simulink model "Taller_2"  (R2025b)
settings: Solver=VariableStepAuto  StartTime=0.0  StopTime=5  RelTol=1e-3
libraries: simulink x7
settings Model: Creator=andre  LastModifiedBy=andre

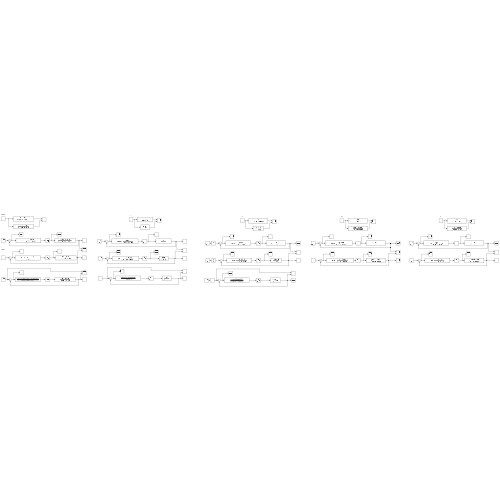
[thumbnail: Simulink's stored preview of the top-level diagram]
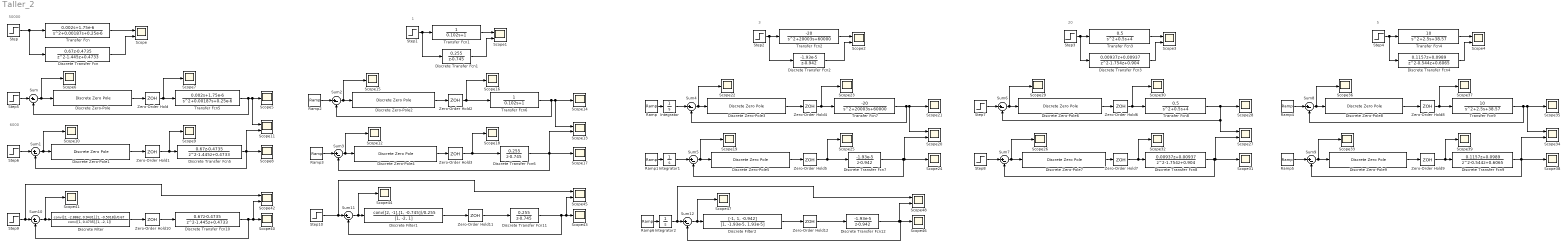
== system Taller_2 ==
  note: 1
  note: 50000
  note: 3
  note: 20
  note: 5
  note: 6000
  Discrete Transfer Fcn : DiscreteTransferFcn  Numerator=[0.67 -0.4735]  Denominator=[1 -1.445 0.4733]
  Discrete Transfer Fcn1 : DiscreteTransferFcn  Numerator=[0.255]  Denominator=[1 -0.745]
  Discrete Transfer Fcn10 : DiscreteTransferFcn  Numerator=[0.67 -0.4735]  Denominator=[1 -1.445 0.4733]
  Discrete Transfer Fcn11 : DiscreteTransferFcn  Numerator=[0.255]  Denominator=[1 -0.745]
  Discrete Transfer Fcn12 : DiscreteTransferFcn  Numerator=[-1.93e-5]  Denominator=[1 -0.942]
  Discrete Transfer Fcn2 : DiscreteTransferFcn  Numerator=[-1.93e-5]  Denominator=[1 -0.942]
  Discrete Transfer Fcn3 : DiscreteTransferFcn  Numerator=[0.00937 0.00937]  Denominator=[1 -1.754 0.904]
  Discrete Transfer Fcn4 : DiscreteTransferFcn  Numerator=[0.1157 0.0989]  Denominator=[1 -0.544 0.6065]
  Discrete Transfer Fcn5 : DiscreteTransferFcn  Numerator=[0.67 -0.4735]  Denominator=[1 -1.445 0.4733]
  Discrete Transfer Fcn6 : DiscreteTransferFcn  Numerator=[0.255]  Denominator=[1 -0.745]
  Discrete Transfer Fcn7 : DiscreteTransferFcn  Numerator=[-1.93e-5]  Denominator=[1 -0.942]
  Discrete Transfer Fcn8 : DiscreteTransferFcn  Numerator=[0.00937 0.00937]  Denominator=[1 -1.754 0.904]
  Discrete Transfer Fcn9 : DiscreteTransferFcn  Numerator=[0.1157 0.0989]  Denominator=[1 -0.544 0.6065]
  Discrete Zero-Pole : DiscreteZeroPole  Zeros=[0.9432 0.9432 0.9432]  Poles=[1 0.7364 0.7364 0.7364]  Gain=3.25e-4  SampleTime=400
  Discrete Zero-Pole1 : DiscreteZeroPole  Zeros=[0.9432 0.9432 0.9432]  Poles=[1 0.7364 0.7364 0.7364]  Gain=3.25e-4  SampleTime=400
  Discrete Zero-Pole2 : DiscreteZeroPole  Zeros=[0.745 0.745 0.745]  Poles=[1 1 0.6749 0.6749 0.6749]  Gain=1.031e-2  SampleTime=0.05
  Discrete Zero-Pole3 : DiscreteZeroPole  Zeros=[0.942 0.942 0.942]  Poles=[1 1 1 0.936 0.936 0.936]  Gain=-0.0433  SampleTime=0.02
  Discrete Zero-Pole4 : DiscreteZeroPole  Zeros=[0.745 0.745 0.745]  Poles=[1 1 0.6749 0.6749 0.6749]  Gain=1.031e-2  SampleTime=0.05
  Discrete Zero-Pole5 : DiscreteZeroPole  Zeros=[0.942 0.942 0.942]  Poles=[1 1 1 0.936 0.936 0.936]  Gain=-0.0433  SampleTime=0.02
  Discrete Zero-Pole6 : DiscreteZeroPole  Zeros=[0.9549 0.9549 0.9549]  Poles=[1 1 0.9581 0.9581 0.9581]  Gain=0.01468  SampleTime=0.2
  Discrete Zero-Pole7 : DiscreteZeroPole  Zeros=[0.9549 0.9549 0.9549]  Poles=[1 1 0.9581 0.9581 0.9581]  Gain=0.01468  SampleTime=0.2
  Discrete Zero-Pole8 : DiscreteZeroPole  Zeros=[0.717 0.717]  Poles=[1 1 0.952 0.952]  Gain=3.75  SampleTime=0.2
  Discrete Zero-Pole9 : DiscreteZeroPole  Zeros=[0.717 0.717]  Poles=[1 1 0.952 0.952]  Gain=3.75  SampleTime=0.2
  Discrete Filter : DiscreteFilter  Numerator=conv([2, -2.8862, 0.9431],[1, -0.5018])/0.67  Denominator=conv([1, 0.4735],[1, -2, 1])
  Discrete Filter1 : DiscreteFilter  Numerator=conv([2, -1],[1, -0.745])/0.255  Denominator=[1, -2, 1]
  Discrete Filter2 : DiscreteFilter  Numerator=[-1, 1, -0.942]  Denominator=[1, -1.93e-5, 1.93e-5]
  Integrator : Integrator
  Integrator1 : Integrator
  Integrator2 : Integrator
  Ramp{,1..6} (7 alike) : simulink/Sources/Ramp  slope=1  start=0  InitialOutput=0
  Scope{,1..4,11,13,20,27,34,42,45,48} (13 alike) : Scope  NumInputPorts=2
      Scope settings: ActiveDisplayYMinimum=-0.87443172150614323  ActiveDisplayYMaximum=7.8698854935552909
      Scope1 settings: ActiveDisplayYMinimum=-0.12499999999997945  ActiveDisplayYMaximum=1.1249999999998153
      Scope11 settings: ActiveDisplayYMinimum=-1  ActiveDisplayYMaximum=1  DataLoggingVariableName=ScopeData11
      Scope13 settings: ActiveDisplayYMinimum=-1  ActiveDisplayYMaximum=1  DataLoggingVariableName=ScopeData13
      Scope2 settings: ActiveDisplayYMinimum=-0.0003749537356942865  ActiveDisplayYMaximum=4.1661526188254047E-5  DataLoggingVariableName=ScopeData2
      Scope20 settings: ActiveDisplayYMinimum=-1  ActiveDisplayYMaximum=1  DataLoggingVariableName=ScopeData20
      Scope27 settings: ActiveDisplayYMinimum=-1  ActiveDisplayYMaximum=1  DataLoggingVariableName=ScopeData27
      Scope3 settings: ActiveDisplayYMinimum=-0.026140229104854404  ActiveDisplayYMaximum=0.2352620619436897  DataLoggingVariableName=ScopeData3
      Scope34 settings: ActiveDisplayYMinimum=-16759.782546183404  ActiveDisplayYMaximum=10006.031814391354  DataLoggingVariableName=ScopeData34
      Scope4 settings: ActiveDisplayYMinimum=-0.049373131397526727  ActiveDisplayYMaximum=0.44435818257774068  DataLoggingVariableName=ScopeData4
      Scope42 settings: ActiveDisplayYMinimum=-11114.4553559121  ActiveDisplayYMaximum=19001.265185022872  DataLoggingVariableName=ScopeData42
      Scope45 settings: ActiveDisplayYMinimum=-2.5344855037279E+9  ActiveDisplayYMaximum=9.5632271965801024E+8  DataLoggingVariableName=ScopeData45
      Scope48 settings: ActiveDisplayYMinimum=-0.56305934372930366  ActiveDisplayYMaximum=5.0675340935637339  DataLoggingVariableName=ScopeData48
  Scope{5..10,12,14..19,21..26,28..33,35..41,43..44,46..47} (36 alike) : Scope
      Scope10 settings: DataLoggingVariableName=ScopeData10
      Scope12 settings: ActiveDisplayYMinimum=-1  ActiveDisplayYMaximum=1  DataLoggingVariableName=ScopeData12
      Scope14 settings: ActiveDisplayYMinimum=-1  ActiveDisplayYMaximum=1  DataLoggingVariableName=ScopeData14
      Scope15 settings: ActiveDisplayYMinimum=-0.11913455922896504  ActiveDisplayYMaximum=1.0722110330606855  DataLoggingVariableName=ScopeData15
      Scope16 settings: ActiveDisplayYMinimum=-1  ActiveDisplayYMaximum=1  DataLoggingVariableName=ScopeData16
      Scope17 settings: ActiveDisplayYMinimum=-1  ActiveDisplayYMaximum=1  DataLoggingVariableName=ScopeData17
      Scope18 settings: ActiveDisplayYMinimum=-1  ActiveDisplayYMaximum=1  DataLoggingVariableName=ScopeData18
      Scope19 settings: ActiveDisplayYMinimum=-1  ActiveDisplayYMaximum=1  DataLoggingVariableName=ScopeData19
      Scope21 settings: ActiveDisplayYMinimum=-1  ActiveDisplayYMaximum=1  DataLoggingVariableName=ScopeData21
      Scope22 settings: ActiveDisplayYMinimum=-1  ActiveDisplayYMaximum=1  DataLoggingVariableName=ScopeData22
      Scope23 settings: ActiveDisplayYMinimum=-1  ActiveDisplayYMaximum=1  DataLoggingVariableName=ScopeData23
      Scope24 settings: ActiveDisplayYMinimum=-1  ActiveDisplayYMaximum=1  DataLoggingVariableName=ScopeData24
      Scope25 settings: ActiveDisplayYMinimum=-1  ActiveDisplayYMaximum=1  DataLoggingVariableName=ScopeData25
      Scope26 settings: ActiveDisplayYMinimum=-1.1632353626194667  ActiveDisplayYMaximum=10.469118263575202  DataLoggingVariableName=ScopeData26
      Scope28 settings: ActiveDisplayYMinimum=-7.3434503553882573  ActiveDisplayYMaximum=11.734447850973403  DataLoggingVariableName=ScopeData28
      Scope29 settings: ActiveDisplayYMinimum=-1  ActiveDisplayYMaximum=1  DataLoggingVariableName=ScopeData29
      Scope30 settings: ActiveDisplayYMinimum=-1  ActiveDisplayYMaximum=1  DataLoggingVariableName=ScopeData30
      Scope31 settings: ActiveDisplayYMinimum=-1  ActiveDisplayYMaximum=1  DataLoggingVariableName=ScopeData31
      Scope32 settings: ActiveDisplayYMinimum=-2660.345058918731  ActiveDisplayYMaximum=23943.105530268582  DataLoggingVariableName=ScopeData32
      Scope33 settings: ActiveDisplayYMinimum=-6005.6817208247221  ActiveDisplayYMaximum=976.6617763905931  DataLoggingVariableName=ScopeData33
      Scope35 settings: ActiveDisplayYMinimum=-1  ActiveDisplayYMaximum=1  DataLoggingVariableName=ScopeData35
      Scope36 settings: ActiveDisplayYMinimum=-1  ActiveDisplayYMaximum=1  DataLoggingVariableName=ScopeData36
      Scope37 settings: ActiveDisplayYMinimum=-1  ActiveDisplayYMaximum=1  DataLoggingVariableName=ScopeData37
      Scope38 settings: ActiveDisplayYMinimum=-973.32427639059324  ActiveDisplayYMaximum=6010.6442208247227  DataLoggingVariableName=ScopeData38
      Scope39 settings: ActiveDisplayYMinimum=-2660.345058918731  ActiveDisplayYMaximum=23943.105530268582  DataLoggingVariableName=ScopeData39
      Scope40 settings: ActiveDisplayYMinimum=-1  ActiveDisplayYMaximum=1  DataLoggingVariableName=ScopeData40
      Scope41 settings: DataLoggingVariableName=ScopeData41
      Scope43 settings: ActiveDisplayYMinimum=-2.5344855037279E+9  ActiveDisplayYMaximum=9.5632271965801024E+8  DataLoggingVariableName=ScopeData43
      Scope44 settings: ActiveDisplayYMinimum=-9.5632271865801024E+8  ActiveDisplayYMaximum=2.5344855047279E+9  DataLoggingVariableName=ScopeData44
      Scope46 settings: ActiveDisplayYMinimum=-0.00013849809070554233  ActiveDisplayYMaximum=0.0012464828163498813  DataLoggingVariableName=ScopeData46
      Scope47 settings: ActiveDisplayYMinimum=-0.56292084563859812  ActiveDisplayYMaximum=5.0662876107473842  DataLoggingVariableName=ScopeData47
      Scope5 settings: ActiveDisplayYMinimum=-1  ActiveDisplayYMaximum=1  DataLoggingVariableName=ScopeData5
      Scope6 settings: ActiveDisplayYMinimum=-1  ActiveDisplayYMaximum=1  DataLoggingVariableName=ScopeData6
      Scope7 settings: ActiveDisplayYMinimum=-1  ActiveDisplayYMaximum=1  DataLoggingVariableName=ScopeData7
      Scope8 settings: ActiveDisplayYMinimum=-1  ActiveDisplayYMaximum=1  DataLoggingVariableName=ScopeData8
      Scope9 settings: ActiveDisplayYMinimum=-1  ActiveDisplayYMaximum=1  DataLoggingVariableName=ScopeData9
  Step{,1..10} (11 alike) : Step  Time=0  SampleTime=0
  Sum{,1..12} (13 alike) : Sum  Inputs=|+-
  Transfer Fcn : TransferFcn  Numerator=[0.002 1.75e-6]  Denominator=[1 0.00187 0.25e-6]
  Transfer Fcn1 : TransferFcn  Denominator=[0.102 1]
  Transfer Fcn2 : TransferFcn  Numerator=[-20]  Denominator=[1 20003 60000]
  Transfer Fcn3 : TransferFcn  Numerator=[0.5]  Denominator=[1 0.5 4]
  Transfer Fcn4 : TransferFcn  Numerator=[10]  Denominator=[1 2.5 38.57]
  Transfer Fcn5 : TransferFcn  Numerator=[0.002 1.75e-6]  Denominator=[1 0.00187 0.25e-6]
  Transfer Fcn6 : TransferFcn  Denominator=[0.102 1]
  Transfer Fcn7 : TransferFcn  Numerator=[-20]  Denominator=[1 20003 60000]
  Transfer Fcn8 : TransferFcn  Numerator=[0.5]  Denominator=[1 0.5 4]
  Transfer Fcn9 : TransferFcn  Numerator=[10]  Denominator=[1 2.5 38.57]
  Zero-Order Hold : ZeroOrderHold  SampleTime=400
  Zero-Order Hold1 : ZeroOrderHold  SampleTime=400
  Zero-Order Hold10 : ZeroOrderHold  SampleTime=400
  Zero-Order Hold11 : ZeroOrderHold  SampleTime=0.03
  Zero-Order Hold12 : ZeroOrderHold  SampleTime=0.02
  Zero-Order Hold2 : ZeroOrderHold  SampleTime=0.05
  Zero-Order Hold3 : ZeroOrderHold  SampleTime=0.05
  Zero-Order Hold4 : ZeroOrderHold  SampleTime=0.02
  Zero-Order Hold5 : ZeroOrderHold  SampleTime=0.02
  Zero-Order Hold{6..9} (4 alike) : ZeroOrderHold  SampleTime=0.2
  wires:
  Transfer Fcn/1 -> Scope/1
  Step/1 -> Discrete Transfer Fcn/1, Transfer Fcn/1
  Transfer Fcn1/1 -> Scope1/1
  Step1/1 -> Discrete Transfer Fcn1/1, Transfer Fcn1/1
  Transfer Fcn2/1 -> Scope2/1
  Step2/1 -> Discrete Transfer Fcn2/1, Transfer Fcn2/1
  Transfer Fcn3/1 -> Scope3/1
  Step3/1 -> Discrete Transfer Fcn3/1, Transfer Fcn3/1
  Step4/1 -> Discrete Transfer Fcn4/1, Transfer Fcn4/1
  Transfer Fcn4/1 -> Scope4/1
  Discrete Transfer Fcn/1 -> Scope/2
  Discrete Transfer Fcn1/1 -> Scope1/2
  Discrete Transfer Fcn2/1 -> Scope2/2
  Discrete Transfer Fcn3/1 -> Scope3/2
  Discrete Transfer Fcn4/1 -> Scope4/2
  Zero-Order Hold/1 -> Scope7/1, Transfer Fcn5/1
  Discrete Zero-Pole/1 -> Zero-Order Hold/1
  Step5/1 -> Sum/1
  Sum/1 -> Scope6/1, Discrete Zero-Pole/1
  Transfer Fcn5/1 -> Scope11/1, Scope5/1, Sum/2
  Discrete Zero-Pole1/1 -> Zero-Order Hold1/1
  Zero-Order Hold1/1 -> Scope9/1, Discrete Transfer Fcn5/1
  Sum1/1 -> Discrete Zero-Pole1/1, Scope10/1
  Step6/1 -> Sum1/1
  Discrete Transfer Fcn5/1 -> Scope8/1, Scope11/2, Sum1/2
  Zero-Order Hold2/1 -> Transfer Fcn6/1, Scope16/1
  Ramp2/1 -> Sum2/1
  Sum3/1 -> Scope12/1, Discrete Zero-Pole4/1
  Zero-Order Hold3/1 -> Discrete Transfer Fcn6/1, Scope18/1
  Discrete Transfer Fcn6/1 -> Scope17/1, Scope13/2, Sum3/2
  Sum2/1 -> Scope15/1, Discrete Zero-Pole2/1
  Transfer Fcn6/1 -> Scope13/1, Scope14/1, Sum2/2
  Discrete Zero-Pole2/1 -> Zero-Order Hold2/1
  Discrete Zero-Pole4/1 -> Zero-Order Hold3/1
  Discrete Zero-Pole5/1 -> Zero-Order Hold5/1
  Transfer Fcn7/1 -> Scope20/1, Scope21/1, Sum4/2
  Integrator/1 -> Sum4/1
  Zero-Order Hold4/1 -> Transfer Fcn7/1, Scope23/1
  Sum5/1 -> Discrete Zero-Pole5/1, Scope19/1
  Zero-Order Hold5/1 -> Discrete Transfer Fcn7/1, Scope25/1
  Integrator1/1 -> Sum5/1
  Discrete Zero-Pole3/1 -> Zero-Order Hold4/1
  Sum4/1 -> Scope22/1, Discrete Zero-Pole3/1
  Discrete Transfer Fcn7/1 -> Scope24/1, Scope20/2, Sum5/2
  Ramp/1 -> Integrator/1
  Ramp1/1 -> Integrator1/1
  Sum6/1 -> Scope29/1, Discrete Zero-Pole6/1
  Zero-Order Hold6/1 -> Transfer Fcn8/1, Scope30/1
  Discrete Zero-Pole6/1 -> Zero-Order Hold6/1
  Discrete Transfer Fcn8/1 -> Scope31/1, Scope27/2, Sum7/2
  Sum7/1 -> Scope26/1, Discrete Zero-Pole7/1
  Zero-Order Hold7/1 -> Scope32/1, Discrete Transfer Fcn8/1
  Discrete Zero-Pole7/1 -> Zero-Order Hold7/1
  Transfer Fcn8/1 -> Sum6/2, Scope27/1, Scope28/1
  Step8/1 -> Sum7/1
  Step7/1 -> Sum6/1
  Sum9/1 -> Discrete Zero-Pole9/1, Scope33/1
  Zero-Order Hold9/1 -> Discrete Transfer Fcn9/1, Scope39/1
  Discrete Zero-Pole8/1 -> Zero-Order Hold8/1
  Sum8/1 -> Scope36/1, Discrete Zero-Pole8/1
  Zero-Order Hold8/1 -> Transfer Fcn9/1, Scope37/1
  Discrete Zero-Pole9/1 -> Zero-Order Hold9/1
  Ramp5/1 -> Sum9/1
  Discrete Transfer Fcn9/1 -> Scope38/1, Scope34/2, Sum9/2
  Ramp4/1 -> Sum8/1
  Transfer Fcn9/1 -> Scope34/1, Scope35/1, Sum8/2
  Discrete Filter/1 -> Zero-Order Hold10/1
  Zero-Order Hold10/1 -> Discrete Transfer Fcn10/1
  Sum10/1 -> Scope41/1, Discrete Filter/1
  Step9/1 -> Scope42/1, Sum10/1
  Discrete Transfer Fcn10/1 -> Scope42/2, Scope40/1, Sum10/2
  Discrete Transfer Fcn11/1 -> Scope45/2, Scope43/1, Sum11/2
  Sum11/1 -> Scope44/1, Discrete Filter1/1
  Step10/1 -> Scope45/1, Sum11/1
  Zero-Order Hold11/1 -> Discrete Transfer Fcn11/1
  Discrete Filter1/1 -> Zero-Order Hold11/1
  Ramp3/1 -> Sum3/1
  Sum12/1 -> Scope47/1, Discrete Filter2/1
  Discrete Filter2/1 -> Zero-Order Hold12/1
  Discrete Transfer Fcn12/1 -> Scope48/2, Scope46/1, Sum12/2
  Integrator2/1 -> Scope48/1, Sum12/1
  Zero-Order Hold12/1 -> Discrete Transfer Fcn12/1
  Ramp6/1 -> Integrator2/1
